simulink model "mock2dev_out"  (R2017b)
settings: Solver=VariableStepAuto  StartTime=0.0  StopTime=10  RelTol=1e-3
model workspace (MAT data in the model file):
  Ts = Simulink.Parameter
  Ts.Value = 0.5
  Ts.DataType = 'auto'
  Ts.Dimensions = [1 1]
libraries: lib_ed247 x1
settings Model: Creator=odufour  LastModifiedBy=odufour
settings DataIOCC: InspectSignalLogs=on
settings CodeAppCC: StateflowObjectComments=on

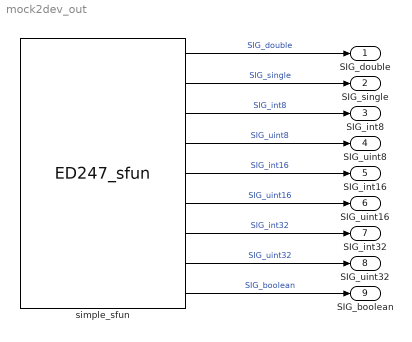
== system mock2dev_out ==
  simple_sfun : lib_ed247/ED247_sfun  configurationFilename='a429_uc_1_simple.xml'  enableLog=off  logFilename=''
      settings: SourceProductName=Airbus ED247
  SIG_double : Outport  SampleTime=Ts
  SIG_single : Outport  Port=2  SampleTime=Ts
  SIG_int8 : Outport  Port=3  SampleTime=Ts
  SIG_uint8 : Outport  Port=4  SampleTime=Ts
  SIG_int16 : Outport  Port=5  SampleTime=Ts
  SIG_uint16 : Outport  Port=6  SampleTime=Ts
  SIG_int32 : Outport  Port=7  SampleTime=Ts
  SIG_uint32 : Outport  Port=8  SampleTime=Ts
  SIG_boolean : Outport  Port=9  SampleTime=Ts
  wires:
  simple_sfun/1 -> SIG_double/1  "SIG_double"
  simple_sfun/2 -> SIG_single/1  "SIG_single"
  simple_sfun/3 -> SIG_int8/1  "SIG_int8"
  simple_sfun/4 -> SIG_uint8/1  "SIG_uint8"
  simple_sfun/5 -> SIG_int16/1  "SIG_int16"
  simple_sfun/6 -> SIG_uint16/1  "SIG_uint16"
  simple_sfun/7 -> SIG_int32/1  "SIG_int32"
  simple_sfun/8 -> SIG_uint32/1  "SIG_uint32"
  simple_sfun/9 -> SIG_boolean/1  "SIG_boolean"
